simulink model "model21"  (R2015a)
settings: Solver=ode3  StartTime=0.0  StopTime=5  RelTol=1e-3
libraries: legoev3lib x4, simulink x1
settings Model: SimulationMode=external  ExtModeTrigDuration=2  Creator=Keshav  LastModifiedBy=Shobhit
settings SolverCC: PositivePriorityOrder=on
settings OptimizationCC: OptimizeModelRefInitCode=on  LifeSpan=1  MaxStackSize=64
settings DebuggingCC: UnderspecifiedInitializationDetection=Classic  MergeDetectMultiDrivingBlocksExec=none  ParameterTunabilityLossMsg=error
settings HardwareCC: ProdLargestAtomicInteger=Long  ProdLargestAtomicFloat=Float  ProdIntDivRoundTo=Zero  ProdEndianess=LittleEndian  ProdHWDeviceType=ARM Compatible->ARM 9
settings RTWCC: SystemTargetFile=ert.tlc  TemplateMakefile=ert_default_tmf  Description=Embedded Coder  GenerateReport=on  RTWVerbose=off  IncludeHyperlinkInReport=on  LaunchReport=on  GenerateTraceInfo=on  GenerateTraceReport=on  GenerateTraceReportSl=on  GenerateTraceReportSf=on  GenerateTraceReportEml=on
settings CodeAppCC: ForceParamTrailComments=on  IgnoreCustomStorageClasses=off  OperatorAnnotations=on  SimulinkDataObjDesc=on  SFDataObjDesc=on  MATLABFcnDesc=on  MangleLength=10  InsertBlockDesc=on  MATLABSourceComments=on
settings ERTTargetCC: GenerateSampleERTMain=off  ParMdlRefBuildCompliant=on  CompOptLevelCompliant=on  ConcurrentExecutionCompliant=on  ERTFirstTimeCompliant=on  SupportNonInlinedSFcns=on  ModelStepFunctionPrototypeControlCompliant=on  CPPClassGenCompliant=on  InlinedParameterPlacement=Hierarchical  ConvertIfToSwitch=on  SuppressUnreachableDefaultCases=on

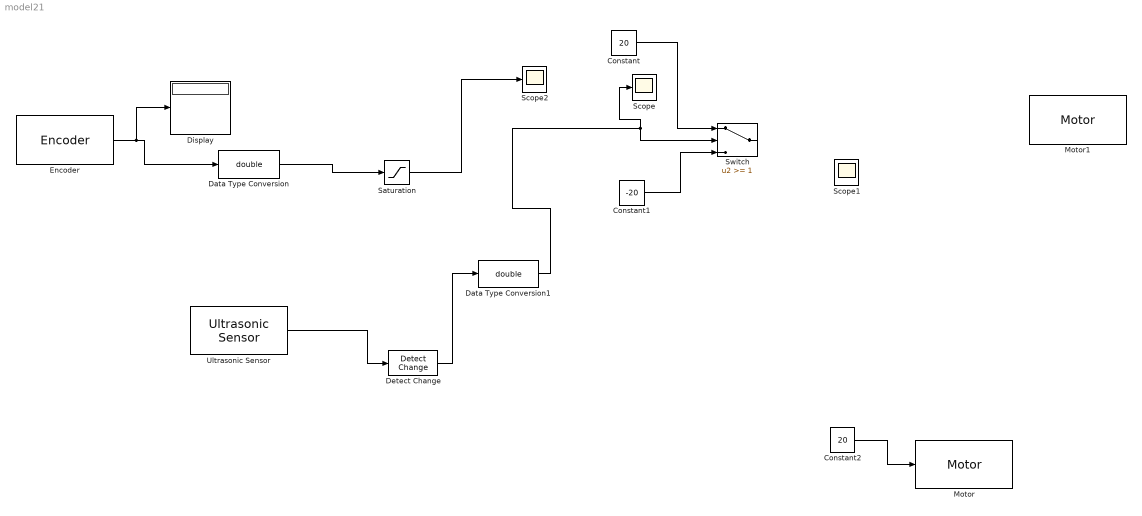
== system model21 ==
  Constant : Constant  Value=20
  Constant1 : Constant  Value=-20
  Constant2 : Constant  Value=20  OutDataTypeStr=int32
  Data Type Conversion : DataTypeConversion  OutDataTypeStr=double
  Data Type Conversion1 : DataTypeConversion  OutDataTypeStr=double
  Detect Change : simulink/Logic and Bit Operations/Detect Change  vinit=0  InputProcessing=Inherited  OutDataTypeStr=boolean
  Display : Display
  Encoder : legoev3lib/Encoder  portNumber=A  opMode=No reset  sampleTime=0.1
  Motor : legoev3lib/Motor  sportNumber=A  sstopAction=Brake
  Motor1 : legoev3lib/Motor  sportNumber=A  sstopAction=Brake
  Saturation : Saturate  UpperLimit=200
  Scope : Scope
      settings: TimeRange=auto  MaxDataPoints=5000  SaveToWorkspace=off  SaveName=ScopeData  YMin=-1.1  YMax=-0.9  SampleTime=-1
  Scope1 : Scope
      settings: TimeRange=auto  MaxDataPoints=5000  SaveToWorkspace=off  YMin=-25.00000  YMax=25.00000  SampleTime=-1
  Scope2 : Scope
      settings: TimeRange=auto  MaxDataPoints=5000  SaveToWorkspace=off  SaveName=ScopeData2  YMin=-1.00000  YMax=1.00000  SampleTime=-1
  Switch : Switch  Threshold=1
  Ultrasonic Sensor : legoev3lib/Ultrasonic Sensor  PortNumber=1  sampleTime=0.1
  wires:
  Constant/1 -> Switch/1
  Constant1/1 -> Switch/3
  Data Type Conversion1/1 -> Switch/2, Scope/1
  Data Type Conversion/1 -> Saturation/1
  Encoder/1 -> Display/1, Data Type Conversion/1
  Constant2/1 -> Motor/1
  Saturation/1 -> Scope2/1
  Ultrasonic Sensor/1 -> Detect Change/1
  Detect Change/1 -> Data Type Conversion1/1
